simulink model "pid_sensor"  (R2023a)
settings: Solver=VariableStepAuto  StartTime=0.0  StopTime=400  RelTol=1e-3
values from neighbouring files (symbols this model uses):
  A1 = 0.0154    [parametros_v1.m]    (also in parametros_v2.m; variables.mat)
  A2 = 5e-5    (= 5e-05)    [parametros_v1.m]    (also in parametros_v2.m; variables.mat)
  az = 0.5    [parametros_v1.m]    (also in parametros_v2.m; variables.mat)
  g = 9.8    [parametros_v1.m]    (also in parametros_v2.m; variables.mat)
  H_max = 0.62    [parametros_v1.m]    (also in parametros_v2.m; variables.mat)
  H_star = 0.31    [parametros_v1.m]    (also in parametros_v2.m; variables.mat)
  kd = 1.07916    [parametros_v2.m]    (also in variables.mat)
  ki = 0.01351    [parametros_v2.m]    (also in variables.mat)
  kp = 0.73979    [parametros_v2.m]    (also in variables.mat)
  N = 0.05171    [parametros_v2.m]    (also in variables.mat)
  Q_star = ro*A2*az*sqrt(2*g*H_star)    [parametros_v1.m]    (also in parametros_v2.m; variables.mat = 0.0616238590158)
  ro = 1000    [parametros_v1.m]    (also in parametros_v2.m; variables.mat)
  semilla = 751    [parametros_v2.m]    (also in variables.mat)
  st = 0.2    [parametros_v2.m]    (also in variables.mat)
libraries: slpidlib x1
settings Model: Creator=emmanuel  LastModifiedBy=empg0
settings OptimizationCC: ReuseModelBlockBuffer=off

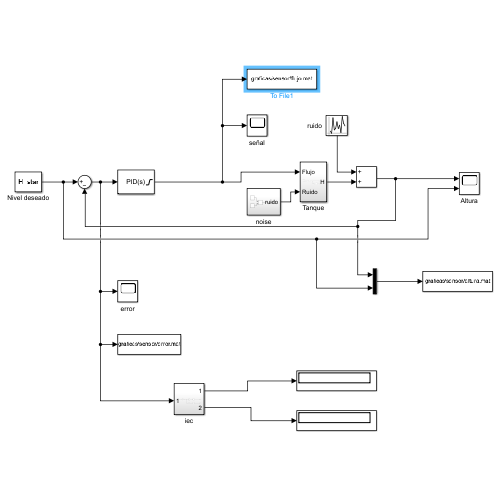
[thumbnail: Simulink's stored preview of the top-level diagram]
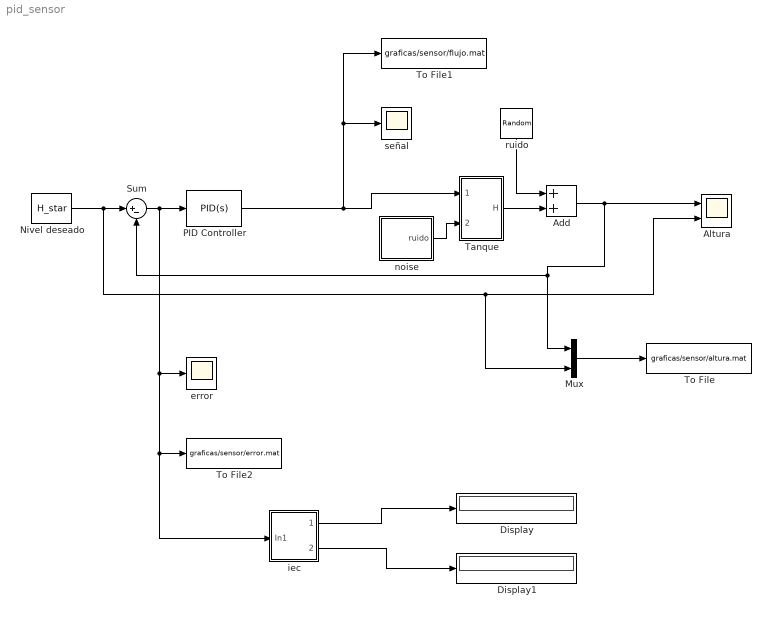
== system pid_sensor ==
  Add : Sum
  Altura : Scope  NumInputPorts=2
  Display : Display
  Display1 : Display
  Mux : Mux  Inputs=2
  Nivel deseado : Constant  Value=H_star
  PID Controller : slpidlib/PID Controller  Controller=PID  Form=Parallel  TimeDomain=Continuous-time  UseExternalTs=off  SampleTime=st  IntegratorMethod=Forward Euler  FilterMethod=Forward Euler  ControllerParametersSource=internal  P=kp  I=ki  UseKiTs=off  D=kd  N=N  UseFilter=on  TunerSelectOption=Frequency Response Based  InitialConditionSource=internal  InitialConditionForIntegrator=0  InitialConditionForFilter=0  DifferentiatorICPrevScaledInput=0  ExternalReset=none  TrackingMode=off  Kt=1  LimitOutput=on  SatLimitsSource=internal  UpperSaturationLimit=0.1  LowerSaturationLimit=0  LinearizeAsGain=off  AntiWindupMode=none  Kb=1  LimitIntegrator=off  UpperIntegratorSaturationLimit=inf  LowerIntegratorSaturationLimit=-inf  POutMin=[]  POutMax=[]  IOutMin=[]  IOutMax=[]  DOutMin=[]  DOutMax=[]  NOutMin=[]  NOutMax=[]  SumOutMin=[]  SumOutMax=[]  SaturationOutMin=[]  SaturationOutMax=[]  PParamMin=[]  PParamMax=[]  IParamMin=[]  IParamMax=[]  DParamMin=[]  DParamMax=[]  NParamMin=[]  NParamMax=[]  KbParamMin=[]  KbParamMax=[]  KtParamMin=[]  KtParamMax=[]  KbOutMin=[]  KbOutMax=[]  KtOutMin=[]  KtOutMax=[]  IntegratorOutMin=[]  IntegratorOutMax=[]  FilterOutMin=[]  FilterOutMax=[]  SumI1OutMin=[]  SumI1OutMax=[]  SumI2OutMin=[]  SumI2OutMax=[]  SumI3OutMin=[]  SumI3OutMax=[]  SumI4OutMin=[]  SumI4OutMax=[]  SumDOutMin=[]  SumDOutMax=[]  DifferentiatorOutMin=[]  DifferentiatorOutMax=[]  FilterDiffOutCoefMin=[]  FilterDiffOutCoefMax=[]  ReciprocalOutMin=[]  ReciprocalOutMax=[]  SumDenOutMin=[]  SumDenOutMax=[]  SumNumOutMin=[]  SumNumOutMax=[]  DivideOutMin=[]  DivideOutMax=[]  UdiffTsProdOutMin=[]  UdiffTsProdOutMax=[]  NTsProdOutMin=[]  NTsProdOutMax=[]  UintegralTsProdOutMin=[]  UintegralTsProdOutMax=[]  UngainTsProdOutMin=[]  UngainTsProdOutMax=[]  ClampingZeroOutDataTypeStr=Inherit: Inherit via back propagation  ClampingZeroOutMin=[]  ClampingZeroOutMax=[]  FilterDenConstantOutDataTypeStr=Inherit: Inherit via back propagation  FilterDenConstantOutMin=[]  FilterDenConstantOutMax=[]  PCopyOutDataTypeStr=Inherit: Inherit via back propagation  PCopyOutMin=[]  PCopyOutMax=[]  NCopyOutDataTypeStr=Inherit: Inherit via back propagation  NCopyOutMin=[]  NCopyOutMax=[]  IntegratorContinuousStateAttributes=''  IntegratorStateMustResolveToSignalObject=off  IntegratorRTWStateStorageClass=Auto  FilterContinuousStateAttributes=''  FilterStateMustResolveToSignalObject=off  FilterRTWStateStorageClass=Auto  ParallelPVariant=InternalParameters  IdealPVariant=Disabled  IVariant=InternalParameters  DVariant=InternalParameters  IntegratorVariant=Continuous  SatVariant=Enabled  AWVariant=Passthrough  PCopyVariant=Disabled  TRVariant=Disabled  FdbkBlocksVariant=Forward  IdealPFdbkVariant=Disabled  SatFdbkVariant=Disabled  DerivativeFilterVariant=ContFilter  NVariant=InternalParameters  NCopyVariant=Disabled  FilterICVariant=InternalICsFilter  IntegratorICVariant=InternalICs  ExternalResetVariant=Disabled  TRSumVariant=Passthrough  SumFdbkVariant=Disabled  SumVariant=Sum_PID  TsampFilterVariant=InternalTs  TsampNgainVariant=Passthrough  TsampIntegralVariant=Disabled_SignalSpec  ExternalSaturationOutDataTypeStr=Inherit: Same as second input
      settings: LibrarySourceBlock=simulink/Discrete/Discrete PID Controller
  Sum : Sum  Inputs=|+-
  Tanque : Subsystem
  To File : ToFile  Filename=graficas/sensor/altura.mat  MatrixName=altura  SampleTime=0.5
  To File1 : ToFile  Filename=graficas/sensor/flujo.mat  MatrixName=flujo  SampleTime=0.5
  To File2 : ToFile  Filename=graficas/sensor/error.mat  MatrixName=error  SampleTime=0.5
  error : Scope
  iec : Subsystem
  noise : Subsystem
  ruido : UniformRandomNumber  Minimum=-H_max*0.03  Maximum=H_max*0.03  Seed=semilla  SampleTime=1
  señal : Scope
  wires:
  Nivel deseado/1 -> Mux/2, Altura/2, Sum/1
  Sum/1 -> iec/1(In1), To File2/1, error/1, PID Controller/1
  PID Controller/1 -> Tanque/1(Flujo), To File1/1, señal/1
  iec/1(Out1) -> Display/1
  noise/1(ruido) -> Tanque/2(Ruido)
  Mux/1 -> To File/1
  iec/2(Out2) -> Display1/1
  Tanque/1(H) -> Add/2
  ruido/1 -> Add/1
  Add/1 -> Mux/1, Sum/2, Altura/1

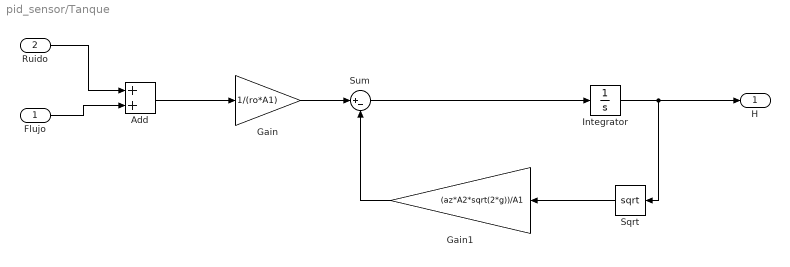
== system pid_sensor/Tanque ==
  Flujo : Inport
  Ruido : Inport  Port=2
  Add : Sum
  Gain : Gain  Gain=1/(ro*A1)
  Gain1 : Gain  Gain=(az*A2*sqrt(2*g))/A1
  Integrator : Integrator  LimitOutput=on  UpperSaturationLimit=0.62  LowerSaturationLimit=0
  Sqrt : Sqrt
  Sum : Sum  Inputs=|+-
  H : Outport
  wires:
  Gain/1 -> Sum/1
  Sum/1 -> Integrator/1
  Sqrt/1 -> Gain1/1
  Gain1/1 -> Sum/2
  Integrator/1 -> H/1, Sqrt/1
  Add/1 -> Gain/1
  Flujo/1 -> Add/2
  Ruido/1 -> Add/1

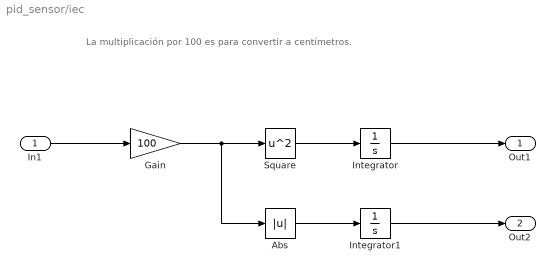
== system pid_sensor/iec ==
  note: La multiplicación por 100 es para convertir a centímetros.
  In1 : Inport
  Abs : Abs  SaturateOnIntegerOverflow=off
  Gain : Gain  Gain=100
  Integrator : Integrator
  Integrator1 : Integrator
  Square : Math  Operator=square  SignedPower=on  RndMeth=Zero
  Out1 : Outport
  Out2 : Outport  Port=2
  wires:
  Square/1 -> Integrator/1
  Integrator/1 -> Out1/1
  In1/1 -> Gain/1
  Gain/1 -> Abs/1, Square/1
  Abs/1 -> Integrator1/1
  Integrator1/1 -> Out2/1

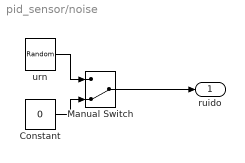
== system pid_sensor/noise ==
  Constant : Constant  Value=0
  Manual Switch : ManualSwitch  CurrentSetting=0
  urn : UniformRandomNumber  Minimum=-Q_star*0.2  Maximum=Q_star*0.2  Seed=140  SampleTime=0.5
  ruido : Outport
  wires:
  urn/1 -> Manual Switch/1
  Constant/1 -> Manual Switch/2
  Manual Switch/1 -> ruido/1
